simulink model "KF_to_play_with_real"  (R2020a)
settings: Solver=FixedStepAuto  StartTime=0.0  StopTime=10.0  FixedStep=0.0001  MaxStep=.001  RelTol=1e-3
values from neighbouring files (symbols this model uses):
  Fes = F-L*H    [KF3_Script.m]    (also in KF_Script.m; LQG_Script.m)
  L = (dlqr(F',H',Q,R))'    [KF3_Script.m]    (also in KF_Script.m; LQG_Script.m)
undefined symbols (not defined in the file or in its folder): G
settings Model: Creator=oboe  LastModifiedBy=Saverio
settings DataIOCC: LimitDataPoints=on  SaveFormat=Array  ReturnWorkspaceOutputs=off
settings OptimizationCC: LifeSpan=inf
settings DebuggingCC: SolverPrmCheckMsg=warning  SFUnexpectedBacktrackingDiag=warning  SFNoUnconditionalDefaultTransitionDiag=warning  SFExecutionAtInitializationDiag=none  ArithmeticOperatorsInVariantConditions=warning
settings HardwareCC: ProdBitPerPointer=32  ProdBitPerSizeT=32  ProdBitPerPtrDiffT=32  ProdLargestAtomicFloat=None  ProdIntDivRoundTo=Undefined  ProdEndianess=Unspecified  ProdWordSize=32  ProdHWDeviceType=32-bit Generic
settings ModelReferenceCC: PropagateSignalLabelsOutOfModel=off
settings SFSimCC: SimUseLocalCustomCode=off  CustomCodeUndefinedFunction=UseInterfaceOnly
settings RTWCC: RTWUseLocalCustomCode=off
settings CodeAppCC: StateflowObjectComments=on
settings GRTTargetCC: TargetLangStandard=C89/C90 (ANSI)
settings ConfigComp: CovMetricSettings=dw  CovHtmlReporting=on  CovSaveCumulativeToWorkspaceVar=on  CovSaveSingleToWorkspaceVar=on  CovExternalEMLEnable=off  CovSFcnEnable=off

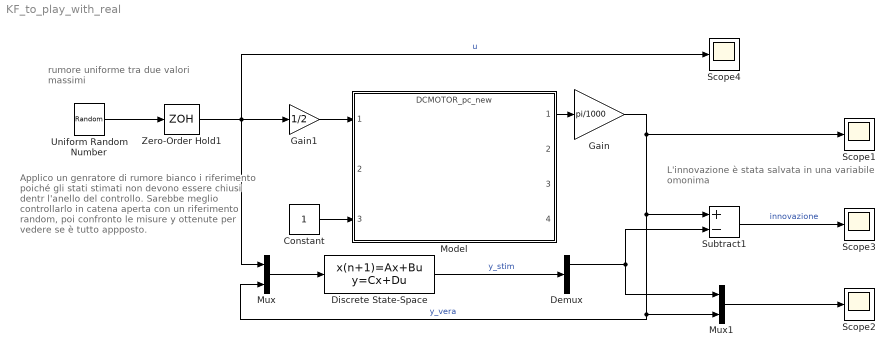
== system KF_to_play_with_real ==
  note: Applico un genratore di rumore bianco i riferimento
      | poiché gli stati stimati non devono essere chiusi dentr
      | l'anello del controllo. Sarebbe meglio controllarlo in catena
      | aperta con un riferimento random, poi confronto le misure y
      | ottenute per vedere se è tutto appposto.
  note: rumore uniforme tra
      | due valori massimi
  note: L'innovazione è stata  salvata in una
      | variabile omonima
  Constant : Constant
  Demux : Demux  Outputs=2
  Discrete State-Space : DiscreteStateSpace  A=Fes  B=[G L]  C=eye(2)  D=zeros(2,2)  SampleTime=.001
  Gain : Gain  Gain=pi/1000
  Gain1 : Gain  Gain=1/2
  Model : ModelReference  ModelNameDialog=DCMOTOR_pc_new.slxp  ModelReferenceVersion=1.21  CopyOfModelProtected=on
  Mux : Mux  Inputs=2
  Mux1 : Mux  Inputs=2
  Scope{1..4} (4 alike) : Scope
  Subtract1 : Sum  Inputs=+-
  Uniform Random Number : UniformRandomNumber  Minimum=-2  Maximum=2  Seed=42  SampleTime=0.001
  Zero-Order Hold1 : ZeroOrderHold  SampleTime=.001
  wires:
  Mux/1 -> Discrete State-Space/1
  Discrete State-Space/1 -> Demux/1  "y_stim"
  Demux/1 -> Subtract1/2, Mux1/1
  Mux1/1 -> Scope2/1
  Subtract1/1 -> Scope3/1  "innovazione"
  Gain/1 -> Mux/2, Mux1/2, Subtract1/1, Scope1/1  "y_vera"
  Uniform Random Number/1 -> Zero-Order Hold1/1
  Zero-Order Hold1/1 -> Gain1/1, Mux/1, Scope4/1  "u"
  Model/1 -> Gain/1
  Constant/1 -> Model/3
  Gain1/1 -> Model/1
